simulink model "task2"  (R2020a)
settings: Solver=VariableStepAuto  StartTime=0.0  StopTime=5  RelTol=1e-3
undefined symbols (not defined in the file): Kd, Kp, p560, qn, R, transl
libraries: roblocks x5
settings Model: Creator=root  LastModifiedBy=root

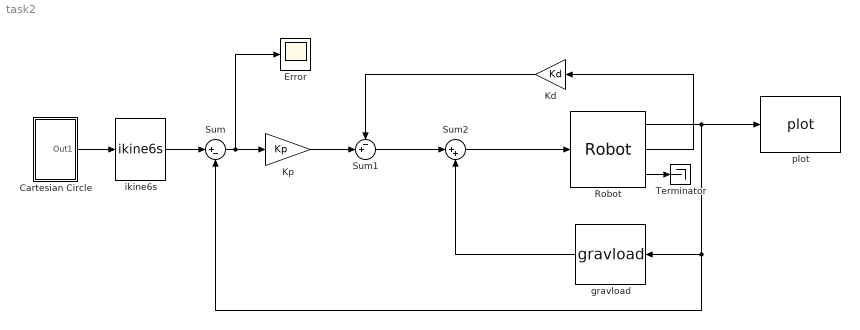
== system task2 ==
  Cartesian Circle : Subsystem
  Error : Scope
  Kd : Gain  Gain=Kd
  Kp : Gain  Gain=Kp
  Robot : roblocks/Arm/Robot  robot=p560.nofriction  q0=[0 0 0 0 0 0]
  Sum : Sum  Inputs=|+-
  Sum1 : Sum  Inputs=-+|
  Sum2 : Sum  Inputs=|++
  Terminator : Terminator
  gravload : roblocks/Arm/gravload  robot=p560.nofriction
  ikine6s : roblocks/Arm/ikine6s  robot=p560.nofriction  conf='luf'
  plot : roblocks/Arm/plot  robot=p560.nofriction  fps=5  holdplot=on
  wires:
  ikine6s/1 -> Sum/1
  Cartesian Circle/1(Out1) -> ikine6s/1
  Robot/2 -> Kd/1
  Sum/1 -> Error/1, Kp/1
  Sum1/1 -> Sum2/1
  Sum2/1 -> Robot/1
  Robot/1 -> plot/1, gravload/1, Sum/2
  gravload/1 -> Sum2/2
  Kp/1 -> Sum1/2
  Kd/1 -> Sum1/1
  Robot/3 -> Terminator/1

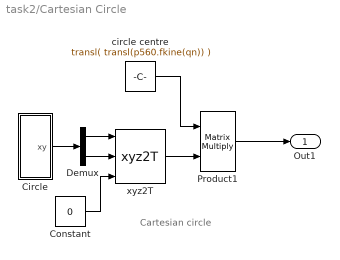
== system task2/Cartesian Circle ==
  note: Cartesian circle
  Circle : Subsystem  mask{radius=R, freq=0.2}
      mask prompts: freq "Frequency (rev/s)"
  Constant : Constant  Value=0
  Demux : Demux  Outputs=2
  Product1 : Product  Multiplication=Matrix(*)  InputSameDT=on  RndMeth=Zero  SaturateOnIntegerOverflow=on  OutDataTypeStr=Inherit: Same as first input
  circle centre : Constant  Value=transl( transl(p560.fkine(qn)) )
  xyz2T : roblocks/Toolbox/xyz2T
  Out1 : Outport
  wires:
  Product1/1 -> Out1/1
  xyz2T/1 -> Product1/2
  circle centre/1 -> Product1/1
  Demux/2 -> xyz2T/2
  Demux/1 -> xyz2T/1
  Constant/1 -> xyz2T/3
  Circle/1(xy) -> Demux/1

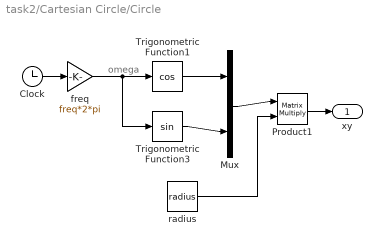
== system task2/Cartesian Circle/Circle ==
  note: omega
  Clock : Clock
  Mux : Mux  Inputs=2
  Product1 : Product  Multiplication=Matrix(*)  RndMeth=Zero
  Trigonometric Function1 : Trigonometry  Operator=cos
  Trigonometric Function3 : Trigonometry
  freq : Gain  Gain=freq*2*pi
  radius : Constant  Value=radius
  xy : Outport
  wires:
  freq/1 -> Trigonometric Function3/1, Trigonometric Function1/1
  Product1/1 -> xy/1
  Clock/1 -> freq/1
  radius/1 -> Product1/2
  Mux/1 -> Product1/1
  Trigonometric Function1/1 -> Mux/1
  Trigonometric Function3/1 -> Mux/2
